simulink model "Test"  (R2021b)
settings: Solver=VariableStepAuto  StartTime=0.0  StopTime=10.0  RelTol=1e-3
undefined symbols (not defined in the file): id, IOSIG_AI_FUEL_IN, NVM_CFG_VEHCLE_MODEL, rte_set_uint8_val, RXSIG_CPD1_FuelMassSignal, SIG_CLASS_COMRX, SIG_CLASS_COMTX, SIG_CLASS_HMI_SND, SIG_CLASS_HMI_TT, SIG_CLASS_IOAL, SIG_CLASS_NVM_CFG, SIG_CLASS_SWC, SIG_CLASS_SYS, SND_FUEL_LEVEL_LOW, SYSSIG_LNN_MODE, SYSSIG_TICK_COUNT, TNC_FuelPrcDisp, TNC_FuelPrcReal, TT_FUEL_LEVEL_LOW, TXSIG_MD_OilPercent, type, val, VEL_VehicleRealSpeed
libraries: simulink x1
(part 2 of 2)

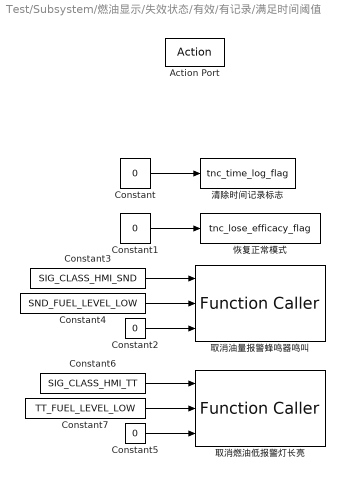
== system Test/Subsystem/燃油显示/失效状态/有效/有记录/满足时间阈值 ==
  Action Port : ActionPort
  Constant{,1..2,5} (4 alike) : Constant  Value=0  OutDataTypeStr=uint8
  Constant3 : Constant  Value=SIG_CLASS_HMI_SND  OutDataTypeStr=uint8
  Constant4 : Constant  Value=SND_FUEL_LEVEL_LOW  OutDataTypeStr=uint16
  Constant6 : Constant  Value=SIG_CLASS_HMI_TT  OutDataTypeStr=uint8
  Constant7 : Constant  Value=TT_FUEL_LEVEL_LOW  OutDataTypeStr=uint16
  取消油量报警蜂鸣器鸣叫 : FunctionCaller  FunctionPrototype=rte_set_uint8_val(type,id,val)  InputArgumentSpecifications=uint8(1), uint16(1), uint8(1)  OutputArgumentSpecifications=<Enter example>
  取消燃油低报警灯长亮 : FunctionCaller  FunctionPrototype=rte_set_uint8_val(type,id,val)  InputArgumentSpecifications=uint8(1), uint16(1), uint8(1)  OutputArgumentSpecifications=<Enter example>
  恢复正常模式 : DataStoreWrite  DataStoreName=tnc_lose_efficacy_flag  IndexOptions=Index vector (dialog)  Indices=1  OutputSizes=1
  清除时间记录标志 : DataStoreWrite  DataStoreName=tnc_time_log_flag  IndexOptions=Index vector (dialog)  Indices=1  OutputSizes=1
  wires:
  Constant/1 -> 清除时间记录标志/1
  Constant1/1 -> 恢复正常模式/1
  Constant2/1 -> 取消油量报警蜂鸣器鸣叫/3
  Constant6/1 -> 取消燃油低报警灯长亮/1
  Constant7/1 -> 取消燃油低报警灯长亮/2
  Constant4/1 -> 取消油量报警蜂鸣器鸣叫/2
  Constant3/1 -> 取消油量报警蜂鸣器鸣叫/1
  Constant5/1 -> 取消燃油低报警灯长亮/3

== system Test/Subsystem/燃油显示/正常状态/无效/有记录/Subsystem ==
  his : Inport  OutDataTypeStr=uint32
  now : Inport  Port=2  OutDataTypeStr=uint32
  If : If  NumInputs=2  IfExpression=u1 > u2  ElseIfExpressions=u1 < u2
  Merge : Merge  Inputs=3
  历史值大于当前值 : Subsystem  TreatAsAtomicUnit=on
  历史值小于当前值 : Subsystem  TreatAsAtomicUnit=on
  历史值等于当前值 : Subsystem  TreatAsAtomicUnit=on
  time_diff : Outport  OutDataTypeStr=uint32
  wires:
  his/1 -> 历史值小于当前值/1(his), 历史值大于当前值/1(his), If/1
  now/1 -> 历史值小于当前值/2(now), 历史值大于当前值/2(now), If/2
  If/1 -> 历史值大于当前值/Action
  If/2 -> 历史值小于当前值/Action
  If/3 -> 历史值等于当前值/Action
  历史值大于当前值/1(time_diff) -> Merge/1
  历史值小于当前值/1(time_diff) -> Merge/2
  历史值等于当前值/1(time_diff) -> Merge/3
  Merge/1 -> time_diff/1

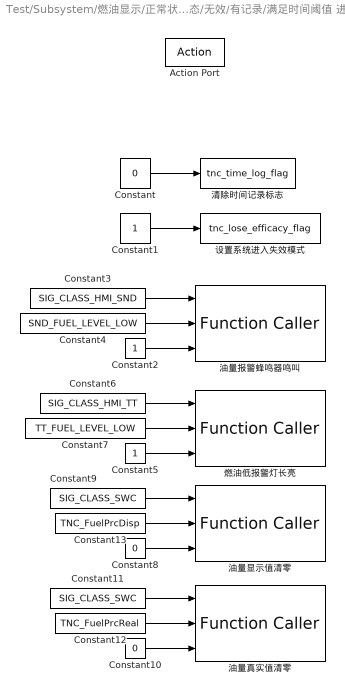
== system Test/Subsystem/燃油显示/正常状态/无效/有记录/满足时间阈值 进入失效模式 时间记录标志复位 ==
  Action Port : ActionPort
  Constant : Constant  Value=0  OutDataTypeStr=uint8
  Constant1 : Constant  OutDataTypeStr=uint8
  Constant10 : Constant  Value=0  OutDataTypeStr=uint8
  Constant11 : Constant  Value=SIG_CLASS_SWC  OutDataTypeStr=uint8
  Constant12 : Constant  Value=TNC_FuelPrcReal  OutDataTypeStr=uint16
  Constant13 : Constant  Value=TNC_FuelPrcDisp  OutDataTypeStr=uint16
  Constant2 : Constant  OutDataTypeStr=uint8
  Constant3 : Constant  Value=SIG_CLASS_HMI_SND  OutDataTypeStr=uint8
  Constant4 : Constant  Value=SND_FUEL_LEVEL_LOW  OutDataTypeStr=uint16
  Constant5 : Constant  OutDataTypeStr=uint8
  Constant6 : Constant  Value=SIG_CLASS_HMI_TT  OutDataTypeStr=uint8
  Constant7 : Constant  Value=TT_FUEL_LEVEL_LOW  OutDataTypeStr=uint16
  Constant8 : Constant  Value=0  OutDataTypeStr=uint8
  Constant9 : Constant  Value=SIG_CLASS_SWC  OutDataTypeStr=uint8
  油量报警蜂鸣器鸣叫 : FunctionCaller  FunctionPrototype=rte_set_uint8_val(type,id,val)  InputArgumentSpecifications=uint8(1), uint16(1), uint8(1)  OutputArgumentSpecifications=<Enter example>
  油量显示值清零 : FunctionCaller  FunctionPrototype=rte_set_uint8_val(type,id,val)  InputArgumentSpecifications=uint8(1), uint16(1), uint8(1)  OutputArgumentSpecifications=<Enter example>
  油量真实值清零 : FunctionCaller  FunctionPrototype=rte_set_uint8_val(type,id,val)  InputArgumentSpecifications=uint8(1), uint16(1), uint8(1)  OutputArgumentSpecifications=<Enter example>
  清除时间记录标志 : DataStoreWrite  DataStoreName=tnc_time_log_flag  IndexOptions=Index vector (dialog)  Indices=1  OutputSizes=1
  燃油低报警灯长亮 : FunctionCaller  FunctionPrototype=rte_set_uint8_val(type,id,val)  InputArgumentSpecifications=uint8(1), uint16(1), uint8(1)  OutputArgumentSpecifications=<Enter example>
  设置系统进入失效模式 : DataStoreWrite  DataStoreName=tnc_lose_efficacy_flag  IndexOptions=Index vector (dialog)  Indices=1  OutputSizes=1
  wires:
  Constant/1 -> 清除时间记录标志/1
  Constant1/1 -> 设置系统进入失效模式/1
  Constant8/1 -> 油量显示值清零/3
  Constant11/1 -> 油量真实值清零/1
  Constant9/1 -> 油量显示值清零/1
  Constant12/1 -> 油量真实值清零/2
  Constant13/1 -> 油量显示值清零/2
  Constant5/1 -> 燃油低报警灯长亮/3
  Constant3/1 -> 油量报警蜂鸣器鸣叫/1
  Constant6/1 -> 燃油低报警灯长亮/1
  Constant10/1 -> 油量真实值清零/3
  Constant4/1 -> 油量报警蜂鸣器鸣叫/2
  Constant7/1 -> 燃油低报警灯长亮/2
  Constant2/1 -> 油量报警蜂鸣器鸣叫/3

== system Test/Subsystem/燃油显示/失效状态/有效/有记录/Subsystem/历史值大于当前值 ==
  his : Inport  OutDataTypeStr=uint32
  now : Inport  Port=2  OutDataTypeStr=uint32
  Action Port : ActionPort
  Add : Sum  Inputs=+-
  Add Constant : Bias  Bias=1
  Add1 : Sum
  Constant : Constant  Value=0xFFFFFFFF  OutDataTypeStr=uint32
  time_diff : Outport  OutDataTypeStr=uint32
  wires:
  Constant/1 -> Add/1
  his/1 -> Add/2
  Add/1 -> Add1/1
  now/1 -> Add1/2
  Add1/1 -> Add Constant/1
  Add Constant/1 -> time_diff/1

== system Test/Subsystem/燃油显示/失效状态/有效/有记录/Subsystem/历史值小于当前值 ==
  his : Inport  OutDataTypeStr=uint32
  now : Inport  Port=2  OutDataTypeStr=uint32
  Action Port : ActionPort
  Add : Sum  Inputs=+-
  time_diff : Outport  OutDataTypeStr=uint32
  wires:
  now/1 -> Add/1
  his/1 -> Add/2
  Add/1 -> time_diff/1

== system Test/Subsystem/燃油显示/失效状态/有效/有记录/Subsystem/历史值等于当前值 ==
  Action Port : ActionPort
  Constant : Constant  Value=0xFFFFFFFF  OutDataTypeStr=uint32
  time_diff : Outport  OutDataTypeStr=uint32
  wires:
  Constant/1 -> time_diff/1

== system Test/Subsystem/燃油显示/正常状态/无效/有记录/Subsystem/历史值大于当前值 ==
  his : Inport  OutDataTypeStr=uint32
  now : Inport  Port=2  OutDataTypeStr=uint32
  Action Port : ActionPort
  Add : Sum  Inputs=+-
  Add Constant : Bias  Bias=1
  Add1 : Sum
  Constant : Constant  Value=0xFFFFFFFF  OutDataTypeStr=uint32
  time_diff : Outport  OutDataTypeStr=uint32
  wires:
  Constant/1 -> Add/1
  his/1 -> Add/2
  Add/1 -> Add1/1
  now/1 -> Add1/2
  Add1/1 -> Add Constant/1
  Add Constant/1 -> time_diff/1

== system Test/Subsystem/燃油显示/正常状态/无效/有记录/Subsystem/历史值小于当前值 ==
  his : Inport  OutDataTypeStr=uint32
  now : Inport  Port=2  OutDataTypeStr=uint32
  Action Port : ActionPort
  Add : Sum  Inputs=+-
  time_diff : Outport  OutDataTypeStr=uint32
  wires:
  now/1 -> Add/1
  his/1 -> Add/2
  Add/1 -> time_diff/1

== system Test/Subsystem/燃油显示/正常状态/无效/有记录/Subsystem/历史值等于当前值 ==
  Action Port : ActionPort
  Constant : Constant  Value=0xFFFFFFFF  OutDataTypeStr=uint32
  time_diff : Outport  OutDataTypeStr=uint32
  wires:
  Constant/1 -> time_diff/1

== matlab function Test/Subsystem/燃油显示/正常状态/有效/大于等于3km//h/filter_higher_3 ==
  data: spd_bf input single size=1; spd_af output single size=1
function spd_af = filter_higher_3(spd_bf)

persistent filter_buf_higher;
if isempty(filter_buf_higher)
    filter_buf_higher = zeros(1,20,class(spd_bf));
end
%spd_af = zeros(1, class(spd_bf));
%for i = 1 : numel(spd_bf)
filter_buf_higher(2:end) = filter_buf_higher(1:end-1);
filter_buf_higher(1) = spd_bf;
spd_af = single(sum(filter_buf_higher)/numel(filter_buf_higher));

== matlab function Test/Subsystem/燃油显示/正常状态/有效/小于3km//h1/filter_lower_3 ==
  data: spd_bf input single size=1; spd_af output single
function spd_af = filter_lower_3(spd_bf)

persistent filter_buf_lower;
if isempty(filter_buf_lower)
    filter_buf_lower = zeros(1, 16, class(spd_bf));
end
%spd_af = zeros(1, class(spd_bf));

filter_buf_lower(2:end) = filter_buf_lower(1:end-1);
filter_buf_lower(1) = spd_bf;
spd_af = single(sum(filter_buf_lower)/numel(filter_buf_lower));
